simulink model "CAPSM_System_IEEE39_260305_110557"  (R2025b)
settings: Solver=ode45  StartTime=0  StopTime=10  MaxStep=0.001  RelTol=1e-3  AbsTol=1e-4
settings Model: Creator=mtk17  LastModifiedBy=mtk17

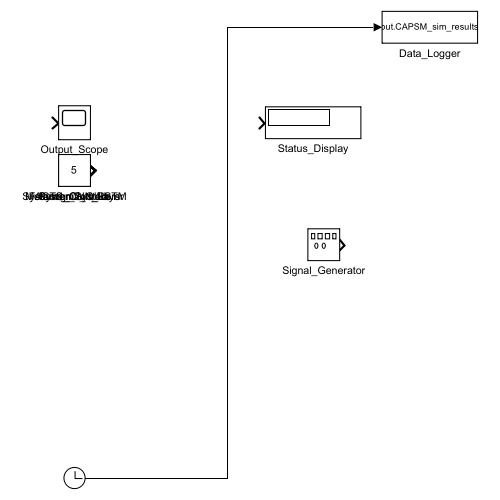
[thumbnail: Simulink's stored preview of the top-level diagram]
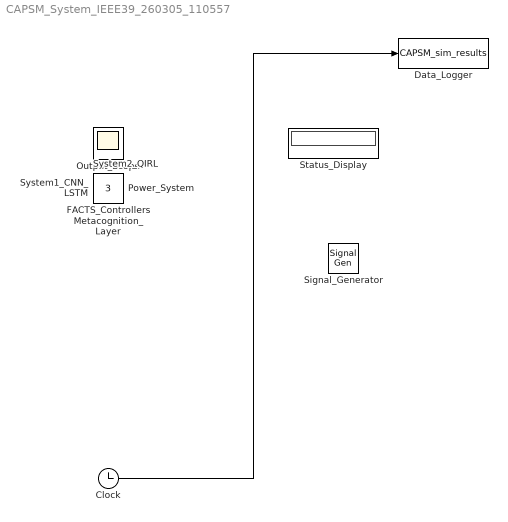
== system CAPSM_System_IEEE39_260305_110557 ==
  Clock : Clock
  Data_Logger : ToWorkspace  VariableName=CAPSM_sim_results  SaveFormat=Timeseries  SampleTime=-1
  FACTS_Controllers : Constant  Value=5
  Metacognition_Layer : Constant  Value=4
  Output_Scope : Scope
  Power_System : Constant
  Signal_Generator : SignalGenerator  Units=rad/sec
  Status_Display : Display
  System1_CNN_LSTM : Constant  Value=2
  System2_QIRL : Constant  Value=3
  wires:
  Clock/1 -> Data_Logger/1
